simulink model "Week2_Problem3"  (R2020b)
settings: Solver=VariableStepAuto  StartTime=0.0  StopTime=120  RelTol=1e-3
undefined symbols (not defined in the file or in its folder): b, ki, kp, m
settings Model: DataDictionary=Problem3_data.sldd  Creator=ASUS  LastModifiedBy=ASUS

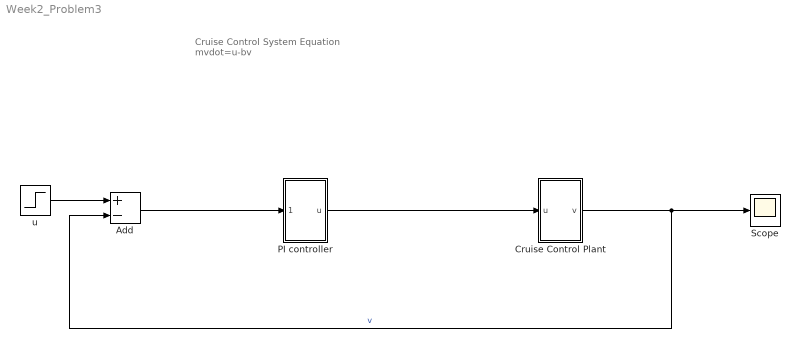
== system Week2_Problem3 ==
  note: Cruise Control System
      |
      | Equation
      | mvdot=u-bv
  Add : Sum  Inputs=+-
  Cruise Control Plant : Subsystem
  PI controller : Subsystem
  Scope : Scope
  u : Step  Time=0  After=u  SampleTime=0
  wires:
  Cruise Control Plant/1(v) -> Scope/1, Add/2  "v"
  u/1 -> Add/1
  Add/1 -> PI controller/1(error)
  PI controller/1(u) -> Cruise Control Plant/1(u)

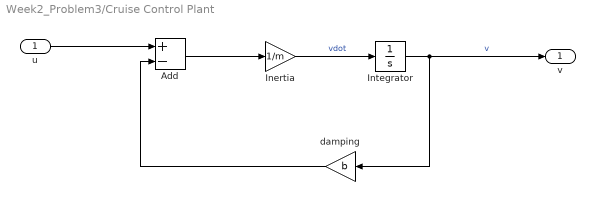
== system Week2_Problem3/Cruise Control Plant ==
  u : Inport
  Add : Sum  Inputs=+-
  Inertia : Gain  Gain=1/m
  Integrator : Integrator
  damping : Gain  Gain=b
  v : Outport
  wires:
  Add/1 -> Inertia/1
  Integrator/1 -> v/1, damping/1  "v"
  u/1 -> Add/1
  damping/1 -> Add/2
  Inertia/1 -> Integrator/1  "vdot"

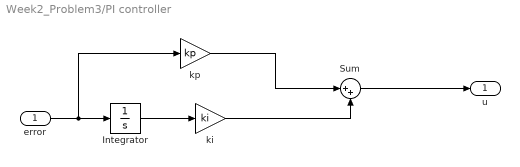
== system Week2_Problem3/PI controller ==
  error : Inport
  Integrator : Integrator
  Sum : Sum  Inputs=|++
  ki : Gain  Gain=ki
  kp : Gain  Gain=kp
  u : Outport
  wires:
  Sum/1 -> u/1
  error/1 -> kp/1, Integrator/1
  kp/1 -> Sum/1
  Integrator/1 -> ki/1
  ki/1 -> Sum/2
